simulink model "ValidateFlyingEvent1"  (R2016b)
settings: Solver=VariableStepAuto  StartTime=0.0  StopTime=10.0  RelTol=1e-3
settings Model: Creator=NEATdemo  LastModifiedBy=NEATdemo

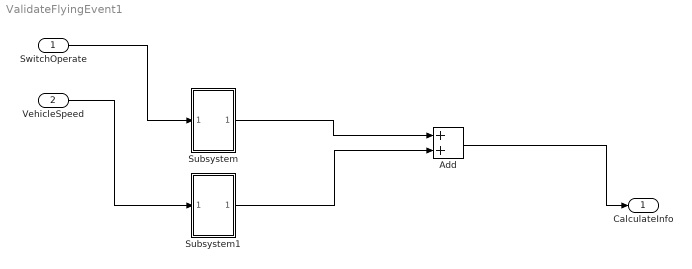
== system ValidateFlyingEvent1 ==
  SwitchOperate : Inport
      settings: AttributesFormatString=SystemSwitch
  VehicleSpeed : Inport  Port=2
      settings: AttributesFormatString=Speed
  Add : Sum
  Subsystem : Subsystem
  Subsystem1 : Subsystem
  CalculateInfo : Outport
  wires:
  SwitchOperate/1 -> Subsystem/1(In1)
  Add/1 -> CalculateInfo/1
  VehicleSpeed/1 -> Subsystem1/1(In1)
  Subsystem/1(Out1) -> Add/1
  Subsystem1/1(Out1) -> Add/2

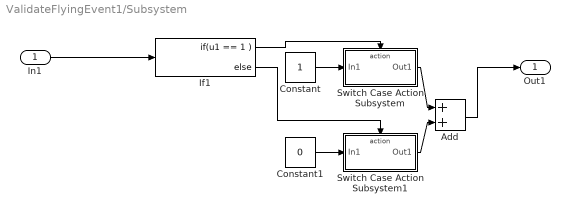
== system ValidateFlyingEvent1/Subsystem ==
  In1 : Inport
  Add : Sum
  Constant : Constant
  Constant1 : Constant  Value=0
  If1 : If  IfExpression=u1 == 1
  Switch Case Action Subsystem : Subsystem  TreatAsAtomicUnit=on
  Switch Case Action Subsystem1 : Subsystem  TreatAsAtomicUnit=on
  Out1 : Outport
  wires:
  Constant1/1 -> Switch Case Action Subsystem1/1(In1)
  Switch Case Action Subsystem/1(Out1) -> Add/1
  In1/1 -> If1/1
  Constant/1 -> Switch Case Action Subsystem/1(In1)
  Switch Case Action Subsystem1/1(Out1) -> Add/2
  If1/1 -> Switch Case Action Subsystem/Action
  Add/1 -> Out1/1
  If1/2 -> Switch Case Action Subsystem1/Action

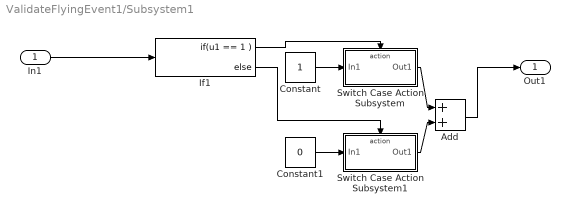
== system ValidateFlyingEvent1/Subsystem1 ==
  In1 : Inport
  Add : Sum
  Constant : Constant
  Constant1 : Constant  Value=0
  If1 : If  IfExpression=u1 == 1
  Switch Case Action Subsystem : Subsystem  TreatAsAtomicUnit=on
  Switch Case Action Subsystem1 : Subsystem  TreatAsAtomicUnit=on
  Out1 : Outport
  wires:
  Constant1/1 -> Switch Case Action Subsystem1/1(In1)
  Switch Case Action Subsystem/1(Out1) -> Add/1
  In1/1 -> If1/1
  Constant/1 -> Switch Case Action Subsystem/1(In1)
  Switch Case Action Subsystem1/1(Out1) -> Add/2
  If1/1 -> Switch Case Action Subsystem/Action
  Add/1 -> Out1/1
  If1/2 -> Switch Case Action Subsystem1/Action

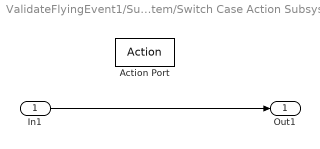
== system ValidateFlyingEvent1/Subsystem/Switch Case Action Subsystem ==
  In1 : Inport
  Action Port : ActionPort
  Out1 : Outport
  wires:
  In1/1 -> Out1/1

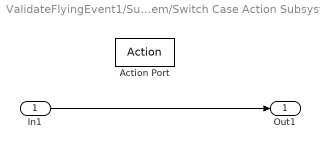
== system ValidateFlyingEvent1/Subsystem/Switch Case Action Subsystem1 ==
  In1 : Inport
  Action Port : ActionPort
  Out1 : Outport
  wires:
  In1/1 -> Out1/1

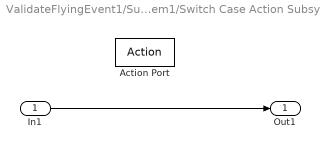
== system ValidateFlyingEvent1/Subsystem1/Switch Case Action Subsystem ==
  In1 : Inport
  Action Port : ActionPort
  Out1 : Outport
  wires:
  In1/1 -> Out1/1

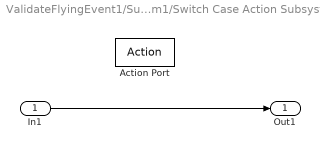
== system ValidateFlyingEvent1/Subsystem1/Switch Case Action Subsystem1 ==
  In1 : Inport
  Action Port : ActionPort
  Out1 : Outport
  wires:
  In1/1 -> Out1/1
